simulink model "arduino_expe"  (R2015a)
settings: Solver=ode3  StartTime=0.0  StopTime=10  FixedStep=0.01  RelTol=1e-3
settings Model: Creator=thomas  LastModifiedBy=thomas

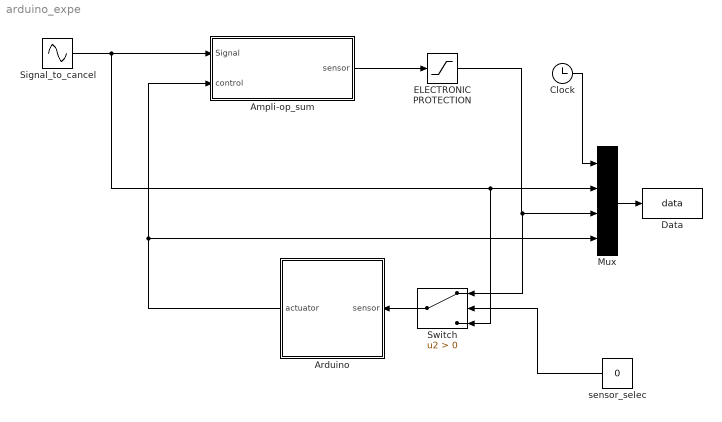
== system arduino_expe ==
  Ampli-op_sum : Subsystem
  Arduino : Subsystem
  Clock : Clock
  Data : ToWorkspace  VariableName=data  SampleTime=-1
  ELECTRONIC PROTECTION : Saturate  UpperLimit=3.3  LowerLimit=0
  Mux : Mux
  Signal_to_cancel : Sin  Bias=1.15  Frequency=6.2832  SampleTime=0.01
  Switch : Switch  Criteria=u2 > Threshold
  sensor_selec : Constant  Value=0
  wires:
  Signal_to_cancel/1 -> Switch/3, Mux/2, Ampli-op_sum/1(Signal)
  Mux/1 -> Data/1
  Clock/1 -> Mux/1
  Arduino/1(actuator) -> Ampli-op_sum/2(control), Mux/4
  Switch/1 -> Arduino/1(sensor)
  sensor_selec/1 -> Switch/2
  Ampli-op_sum/1(sensor) -> ELECTRONIC PROTECTION/1
  ELECTRONIC PROTECTION/1 -> Switch/1, Mux/3

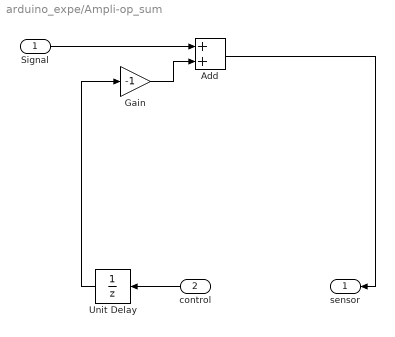
== system arduino_expe/Ampli-op_sum ==
  Signal : Inport
  control : Inport  Port=2
  Add : Sum
  Gain : Gain  Gain=-1
  Unit Delay : UnitDelay  SampleTime=-1
  sensor : Outport
  wires:
  Add/1 -> sensor/1
  Signal/1 -> Add/1
  Gain/1 -> Add/2
  control/1 -> Unit Delay/1
  Unit Delay/1 -> Gain/1

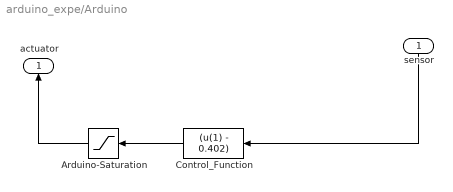
== system arduino_expe/Arduino ==
  sensor : Inport
  Arduino-Saturation : Saturate  UpperLimit=3.3  LowerLimit=0
  Control_Function : Fcn  Expr=(u(1) - 0.402)
  actuator : Outport
  wires:
  Control_Function/1 -> Arduino-Saturation/1
  Arduino-Saturation/1 -> actuator/1
  sensor/1 -> Control_Function/1
